simulink model "problem2Simulink"  (R2023a)
settings: Solver=VariableStepAuto  StartTime=0.0  StopTime=50  RelTol=1e-3
undefined symbols (not defined in the file): A1, a1, A2, a2, g, K
settings Model: Creator=rainsball  LastModifiedBy=rainsball
settings DebuggingCC: AlgebraicLoopMsg=none

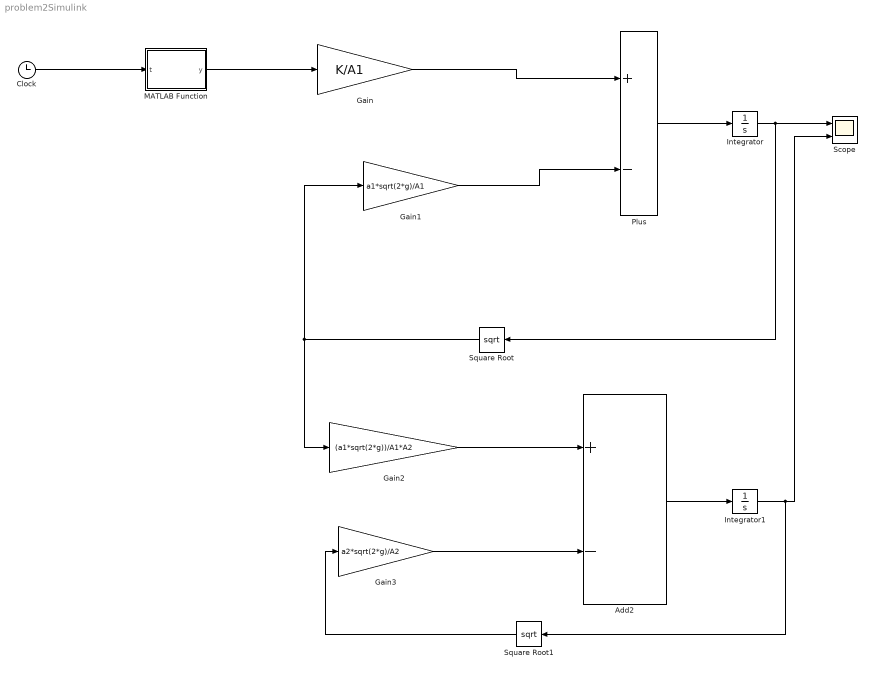
== system problem2Simulink ==
  Add2 : Sum  Inputs=+-
  Clock : Clock
      settings: Decimation=50
  Gain : Gain  Gain=K/A1
  Gain1 : Gain  Gain=a1*sqrt(2*g)/A1
  Gain2 : Gain  Gain=(a1*sqrt(2*g))/A1*A2
  Gain3 : Gain  Gain=a2*sqrt(2*g)/A2
  Integrator : Integrator  InitialCondition=1
  Integrator1 : Integrator
  MATLAB Function : MATLAB Function  TreatAsAtomicUnit=on
  Plus : Sum  Inputs=+-
  Scope : Scope  NumInputPorts=2
  Square Root : Sqrt
  Square Root1 : Sqrt
  wires:
  Gain/1 -> Plus/1
  Gain1/1 -> Plus/2
  Plus/1 -> Integrator/1
  Integrator/1 -> Square Root/1, Scope/1
  Square Root/1 -> Gain2/1, Gain1/1
  Gain2/1 -> Add2/1
  Gain3/1 -> Add2/2
  Add2/1 -> Integrator1/1
  Integrator1/1 -> Square Root1/1, Scope/2
  Square Root1/1 -> Gain3/1
  Clock/1 -> MATLAB Function/1(t)
  MATLAB Function/1(y) -> Gain/1

== matlab function problem2Simulink/MATLAB Function ==
  data: t input; y output
function y = fcn(t)
 y =  1 + 0.1*sin(t);
%y = u;
